simulink model "pendmove2"  (R2015b)
settings: Solver=ode45  StartTime=0.0  StopTime=10  RelTol=1e-3
PreLoadFcn:
  | hwinit
values from neighbouring files (symbols this model uses):
  adingain = [1 1]    [data_pend.mat]    (also in hwinit.m = [1, 1]; matlab.mat)
  adinoffs = [-0.2677 -0.1619]    [data_pend.mat]    (also in hwinit.m = [-0.2769;-0.1613]; matlab.mat = [-0.2732 -0.1636])
  daoutgain = 0.9    [data_pend.mat]    (also in hwinit.m = [0.9]; matlab.mat)
  daoutoffs = 0    [data_pend.mat]    (also in hwinit.m = [0]; matlab.mat)
  h = 0.01    [calib.m]    (also in data_pend.mat; matlab.mat; model.m; nl_pend_dynamics2.m)
undefined symbols (not defined in the file or in its folder): Advantech, PCI
libraries: sldrtlib x2, simulink x1
settings Model: Creator=zhidayat  LastModifiedBy=wvangeest
settings DataIOCC: SaveFormat=Array
settings OptimizationCC: ExpressionDepthLimit=2147483647
settings DebuggingCC: StateNameClashWarn=warning  StrictBusMsg=ErrorOnBusTreatedAsVector
settings HardwareCC: ProdBitPerPointer=32  ProdLargestAtomicFloat=None  ProdIntDivRoundTo=Undefined  ProdEndianess=Unspecified  ProdWordSize=32  ProdHWDeviceType=32-bit Generic
settings GRTTargetCC: GeneratePreprocessorConditionals=Disable all  CombineOutputUpdateFcns=off  GRTInterface=on
settings ConfigComp: CovModelRefEnable=Off

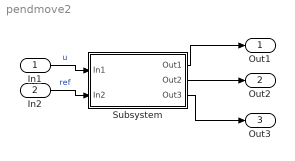
== system pendmove2 ==
  In1 : Inport
  In2 : Inport  Port=2
  Subsystem : Subsystem  StartFcn=hwinit
  Out1 : Outport
  Out2 : Outport  Port=2
  Out3 : Outport  Port=3
  wires:
  In1/1 -> Subsystem/1(In1)  "u"
  In2/1 -> Subsystem/2(In2)  "ref"
  Subsystem/2(Out2) -> Out2/1
  Subsystem/1(Out1) -> Out1/1
  Subsystem/3(Out3) -> Out3/1

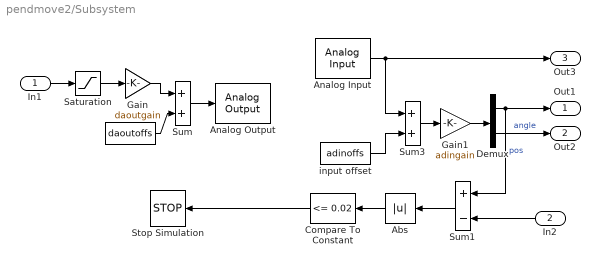
== system pendmove2/Subsystem ==
  In1 : Inport
  In2 : Inport  Port=2
  " " : Constant  Value=daoutoffs
  Abs : Abs
  Analog Input : sldrtlib/Analog Input  SampleTime=h  MaxMissedTicks=ticklost  ShowMissedTicks=off  YieldWhenWaiting=on  DrvName=Advantech/PCI-1711  DrvAddress=4294967295  DrvOptions=zeros(1,0)  Channels=adinchannels  RangeMode=2  VoltRange=1  DataType=1
      settings: AttributesFormatString=Advantech\nPCI-1711 [auto]
  Analog Output : sldrtlib/Analog Output  SampleTime=h  MaxMissedTicks=ticklost  ShowMissedTicks=off  YieldWhenWaiting=off  DrvName=Advantech/PCI-1711  DrvAddress=4294967295  DrvOptions=zeros(1,0)  Channels=daoutchannels  RangeMode=2  VoltRange=2  InitialValue=0  FinalValue=0
      settings: AttributesFormatString=Advantech\nPCI-1711 [auto]
  Compare To Constant : simulink/Logic and Bit Operations/Compare To Constant  relop=<=  const=0.02  OutDataTypeStr=boolean  ZeroCross=off
  Demux : Demux  Outputs=2
  Gain : Gain  Gain=daoutgain  SaturateOnIntegerOverflow=on  OutDataTypeStr=Inherit: Same as input  ParamDataTypeStr=Inherit: Same as input
  Gain1 : Gain  Gain=adingain  SaturateOnIntegerOverflow=on  OutDataTypeStr=Inherit: Same as input  ParamDataTypeStr=Inherit: Same as input
  Saturation : Saturate
  Stop Simulation : Stop
  Sum : Sum  SaturateOnIntegerOverflow=on  InputSameDT=on  OutDataTypeStr=Inherit: Same as first input
  Sum1 : Sum  Inputs=+-
  Sum3 : Sum  SaturateOnIntegerOverflow=on  InputSameDT=on  OutDataTypeStr=Inherit: Same as first input
  input offset : Constant  Value=adinoffs
  Out1 : Outport
  Out2 : Outport  Port=2
  Out3 : Outport  Port=3
  wires:
  " "/1 -> Sum/2
  Gain/1 -> Sum/1
  Sum/1 -> Analog Output/1
  Saturation/1 -> Gain/1
  Gain1/1 -> Demux/1
  Demux/1 -> Out1/1, Sum1/1  "pos"
  input offset/1 -> Sum3/2
  Sum3/1 -> Gain1/1
  Sum1/1 -> Abs/1
  Abs/1 -> Compare To Constant/1
  In1/1 -> Saturation/1
  Demux/2 -> Out2/1  "angle"
  In2/1 -> Sum1/2
  Compare To Constant/1 -> Stop Simulation/1
  Analog Input/1 -> Sum3/1, Out3/1
